simulink subsystem "iLBCTransmit"  (R2024b)
settings: Solver=VariableStepAuto  StartTime=0.0  StopTime=10.0  RelTol=1e-3
values from neighbouring files (symbols this model uses):
  in = pn()    [waveform_generator_Preamble.m]
  LSF = hexToArray(LSF,1)    [Full_transmit.m]
undefined symbols (not defined in the file or in its folder): dspblkCoreblockFVToolHelper, gcbh, ilbc, ilbcMode
libraries: simulink x19, matrix_library x13, dspmtrx3 x9, dspquant2 x6, dspilbclib x5, dspstat3 x5, dspsigops x5, simulink_need_slupdate x2, audiosources x1, dsplp x1, dspsolvers x1
(part 1 of 2)
settings Model: Creator=fredr  LastModifiedBy=fredr

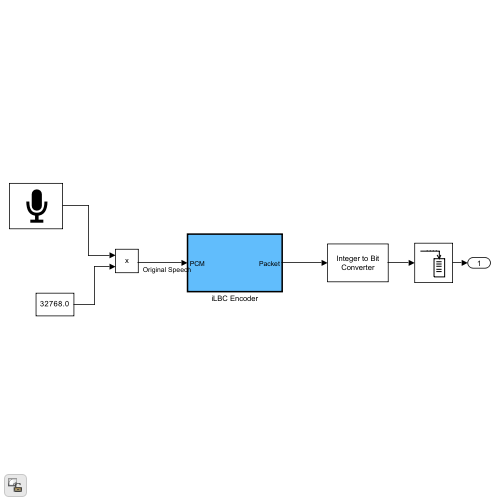
[thumbnail: Simulink's stored preview of the top-level diagram]
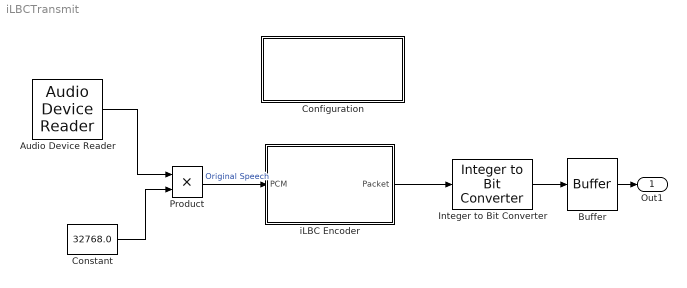
== system iLBCTransmit ==
  Audio Device Reader : audiosources/Audio Device Reader  Driver=DirectSound  Device=Default  SampleRate=8000  NumChannels=1  SamplesPerFrame=240  BitDepth=16-bit integer  NumBuffers=10  DefaultInputChannelMapping=on  InputChannelMapping=1:2  OutputNumOverrunSamples=off  OutputDataType=double  DriverIdx=1  DeviceWarnFlag=''
  Buffer : Buffer  N=200  OutputFrames=off
  Configuration : Subsystem  mask(iLBC Configuration){ilbcDialogMode=13.33 kbit/sec mode, ilbcDialogDatatype=double}
      mask prompts: ilbcDialogMode "iLBC mode:"; ilbcDialogDatatype "Internal data type:"
      mask help:
      | The iLBC standard is defined for two data rates: 13.33 kbit/sec and 15.20 kbit/sec.  Running under 13.33 kbit/sec, the encoder creates and outputs a compressed speech packet every 30ms.  With the 15.20 kbit/sec data rate, the encoder will output a packet every 20ms.  For the 13.33 kbit/sec mode, the packet size is a uint8 column vector of length 50, where each element represents one byte.  For the 15.20 kbit/sec mode, the packet is of length 38 bytes.
      |
      | The "Internal Data Type" option controls the precision for all internal floating point calculations in the iLBC Encoder and Decoder. The possible options are double and single precision.
      mask init:
      | if ilbcDialogMode == 1
      |     ilbcModeStr = '13.33';
      | elseif ilbcDialogMode == 2
      |     ilbcModeStr = '15.20';
      | end
      | 
      | if ilbcDialogDatatype == 1
      |     ilbcDatatype = 'double';
      | elseif ilbcDialogDatatype == 2
      |     ilbcDatatype = 'single';
      | end
      mask TypeOptions ilbcDialogMode: 13.33 kbit/sec mode | 15.20 kbit/sec mode
      mask TypeOptions ilbcDialogDatatype: double | single
      mask Display:
      | disp([ilbcModeStr ' kb/sec mode\n' ...
      |     'Internal data type: ' ilbcDatatype '\n' ...
      |     '[Double-click to change]']);
  Constant : Constant  Value=32768.0
  Integer to Bit Converter : simulink/Logic and Bit Operations/Integer to Bit Converter  nbits=8  signedInputValues=Unsigned  bitOrder=MSB first  outDtype=Inherit via internal rule
  Product : Product  OutDataTypeStr=int16
  iLBC Encoder : Subsystem  TreatAsAtomicUnit=on
  Out1 : Outport
  wires:
  Integer to Bit Converter/1 -> Buffer/1
  Product/1 -> iLBC Encoder/1(PCM)  "Original Speech"
  Audio Device Reader/1 -> Product/1
  iLBC Encoder/1(Packet) -> Integer to Bit Converter/1
  Buffer/1 -> Out1/1
  Constant/1 -> Product/2

== system iLBCTransmit/Configuration ==

== system iLBCTransmit/iLBC Encoder ==
  note: Section 3 of the iLBC standard
  PCM : Inport
  Calculate Residual (3.3) : Subsystem  TreatAsAtomicUnit=on
  Create Packet (3.8) : Subsystem  TreatAsAtomicUnit=on
  Data Type Conversion : DataTypeConversion  OutDataTypeStr=ilbcDatatype  SaturateOnIntegerOverflow=off  RndMeth=Floor
  Encode Data (3.5 - 3.7) : Subsystem  TreatAsAtomicUnit=on
  Encoder LPC Analysis (3.2) : Subsystem  TreatAsAtomicUnit=on
  High Pass (3.1) : DiscreteFilter  LoadFcn=dspblkCoreblockFVToolHelper(gcbh,'load');  Numerator=ilbc.hpi_zero_coefsTbl  Denominator=ilbc.hpi_pole_coefsTbl  InputProcessing=Columns as channels (frame based)  FilterStructure=Direct form II transposed  a0EqualsOne=on  NumAccumDataTypeStr=Inherit: Same as product output  DenAccumDataTypeStr=Inherit: Same as product output
      settings: CopyFcn=dspblkCoreblockFVToolHelper(gcbh,'copy');  DeleteFcn=dspblkCoreblockFVToolHelper(gcbh,'close');  ModelCloseFcn=dspblkCoreblockFVToolHelper(gcbh,'close');  PreSaveFcn=dspblkCoreblockFVToolHelper(gcbh,'presave');  PostSaveFcn=dspblkCoreblockFVToolHelper(gcbh,'postsave');  CloseFcn=dspblkCoreblockFVToolHelper(gcbh,'close');
  Perceptual Weighting (3.4) : dspmtrx3/Array-Vector Multiply  mode=Mute  saveAsFlag=0  Dimension=1  V_Source=Dialog parameter  V_VectFromMask=ilbc.LPC_CHIRP_WEIGHTDENUM.^(0:10)'  roundingMode=Floor  overflowMode=off  firstCoeffSignedness=Auto  firstCoeffDataTypeStr=Inherit: Same word length as input  firstCoeffMin=[]  firstCoeffMax=[]  firstCoeffLastDataTypeStr=Inherit: Same word length as input  prodOutputSignedness=Auto  accumSignedness=Auto  outputSignedness=Auto  outputDataTypeStr=Inherit: Same as product output  outputMin=[]  outputMax=[]  outputLastDataTypeStr=Inherit: Same as product output
  Packet : Outport  VectorParamsAs1DForOutWhenUnconnected=off
  wires:
  Encoder LPC Analysis (3.2)/2(Synthesis Filters) -> Encode Data (3.5 - 3.7)/1(Synthesis), Calculate Residual (3.3)/1(Synthesis Filters)
  Perceptual Weighting (3.4)/1 -> Encode Data (3.5 - 3.7)/2(Weights)
  PCM/1 -> Data Type Conversion/1
  Create Packet (3.8)/1(Packet) -> Packet/1
  Calculate Residual (3.3)/1(Residual) -> Encode Data (3.5 - 3.7)/3(Residual)
  Encoder LPC Analysis (3.2)/3(Weight Filters) -> Perceptual Weighting (3.4)/1
  Encode Data (3.5 - 3.7)/1(Start State Number) -> Create Packet (3.8)/2(Start State Number)
  Encode Data (3.5 - 3.7)/2(State First) -> Create Packet (3.8)/3(State First)
  Encode Data (3.5 - 3.7)/3(Start State Gain Index) -> Create Packet (3.8)/4(Start State Gain Index)
  Encode Data (3.5 - 3.7)/4(Start State Indices) -> Create Packet (3.8)/5(Start State Indices)
  Encode Data (3.5 - 3.7)/5(Code Indices) -> Create Packet (3.8)/6(Code Indices)
  Encode Data (3.5 - 3.7)/6(Gain Indices) -> Create Packet (3.8)/7(Gain Indices)
  High Pass (3.1)/1 -> Encoder LPC Analysis (3.2)/1(Data), Calculate Residual (3.3)/2(Data)
  Encoder LPC Analysis (3.2)/1(LSF Indices) -> Create Packet (3.8)/1(LSF Indices)
  Data Type Conversion/1 -> High Pass (3.1)/1

== system iLBCTransmit/iLBC Encoder/Calculate Residual (3.3) ==
  Synthesis Filters : Inport
  Data : Inport  Port=2
  Assignment1 : Assignment  NumberOfDimensions=2  OutputInitialize=Specify size for each dimension in table  IndexOptions=Assign all,Index vector (port)  Indices=-1,1  OutputSizes=40,ilbc.NSUB{ilbcMode}
  For Iterator : ForIterator  IterationLimit=ilbc.NSUB{ilbcMode}  IterationVariableDataType=int8
  Reshape2 : Reshape  OutputDimensionality=Customize  OutputDimensions=[40 ilbc.NSUB{ilbcMode}]
  Selector1 : Selector  NumberOfDimensions=2  InputPortWidth=3  IndexOptions=Select all,Index vector (port)  Indices=-1,-1  OutputSizes=1
  Selector2 : Selector  NumberOfDimensions=2  InputPortWidth=3  IndexOptions=Select all,Index vector (port)  Indices=-1,-1  OutputSizes=1
  Time-Varying Analysis Filter1 : DiscreteFir  CoefSource=Input port  Coefficients=[1 -.95]  InputProcessing=Columns as channels (frame based)  AccumDataTypeStr=Inherit: Same as product output  OutDataTypeStr=Inherit: Same as input
      settings: InputPortMap=u0,u1
  tp7f274a0e_53ba_403c_9211_c5fc596ffe5e : Math  Operator=transpose  SignedPower=on
  Residual : Outport  VectorParamsAs1DForOutWhenUnconnected=off
  wires:
  tp7f274a0e_53ba_403c_9211_c5fc596ffe5e/1 -> Time-Varying Analysis Filter1/2
  Selector1/1 -> tp7f274a0e_53ba_403c_9211_c5fc596ffe5e/1
  For Iterator/1 -> Assignment1/2, Selector2/2, Selector1/2
  Reshape2/1 -> Selector2/1
  Data/1 -> Reshape2/1
  Synthesis Filters/1 -> Selector1/1
  Assignment1/1 -> Residual/1
  Selector2/1 -> Time-Varying Analysis Filter1/1
  Time-Varying Analysis Filter1/1 -> Assignment1/1

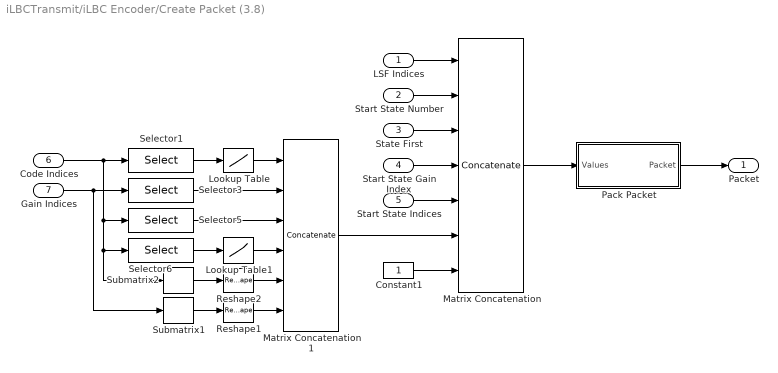
== system iLBCTransmit/iLBC Encoder/Create Packet (3.8) ==
  LSF Indices : Inport
  Start State Number : Inport  Port=2
  State First : Inport  Port=3
  Start State Gain Index : Inport  Port=4
  Start State Indices : Inport  Port=5
  Code Indices : Inport  Port=6
  Gain Indices : Inport  Port=7
  Constant1 : Constant  OutDataTypeStr=uint8
  Lookup Table : Lookup_n-D  NumberOfTableDimensions=1  BreakpointsForDimension1=[0:255]  Table=[0:57 zeros(1,70) 64:121 zeros(1,70)]  ExtrapMethod=Clip
  Lookup Table1 : Lookup_n-D  NumberOfTableDimensions=1  BreakpointsForDimension1=[0:255]  Table=[0:43 zeros(1,64) 44:107 zeros(1,64) 108:127]  ExtrapMethod=Clip
  Matrix Concatenation : Concatenate  NumInputs=7  Mode=Multidimensional array
  Matrix Concatenation1 : Concatenate  NumInputs=6  Mode=Multidimensional array
  Pack Packet : Subsystem  TreatAsAtomicUnit=on
  Reshape1 : Reshape  OutputDimensionality=Column vector (2-D)
  Reshape2 : Reshape  OutputDimensionality=Column vector (2-D)
  Selector1 : Selector  NumberOfDimensions=2  InputPortWidth=3  IndexOptions=Select all,Index vector (dialog)  Indices=-1,1  OutputSizes=1
  Selector3 : Selector  NumberOfDimensions=2  InputPortWidth=3  IndexOptions=Select all,Index vector (dialog)  Indices=-1,1  OutputSizes=1
  Selector5 : Selector  NumberOfDimensions=2  InputPortWidth=3  IndexOptions=Index vector (dialog),Index vector (dialog)  Indices=1,2  OutputSizes=1
  Selector6 : Selector  NumberOfDimensions=2  InputPortWidth=3  IndexOptions=Index vector (dialog),Index vector (dialog)  Indices=2:3,2  OutputSizes=1
  Submatrix1 : matrix_library/Submatrix  RowSpan=All rows  RowStartMode=First  RowStartIndex=1  RowEndMode=Last  RowEndIndex=1  ColSpan=Range of columns  ColStartMode=Index  ColStartIndex=2  ColEndMode=Last  ColEndIndex=1
  Submatrix2 : matrix_library/Submatrix  RowSpan=All rows  RowStartMode=First  RowStartIndex=1  RowEndMode=Last  RowEndIndex=1  ColSpan=Range of columns  ColStartMode=Index  ColStartIndex=3  ColEndMode=Last  ColEndIndex=1
  Packet : Outport  VectorParamsAs1DForOutWhenUnconnected=off
  wires:
  LSF Indices/1 -> Matrix Concatenation/1
  Start State Number/1 -> Matrix Concatenation/2
  State First/1 -> Matrix Concatenation/3
  Start State Gain Index/1 -> Matrix Concatenation/4
  Start State Indices/1 -> Matrix Concatenation/5
  Constant1/1 -> Matrix Concatenation/7
  Code Indices/1 -> Selector1/1, Selector5/1, Selector6/1, Submatrix2/1
  Selector1/1 -> Lookup Table/1
  Matrix Concatenation1/1 -> Matrix Concatenation/6
  Submatrix1/1 -> Reshape1/1
  Selector6/1 -> Lookup Table1/1
  Selector5/1 -> Matrix Concatenation1/3
  Submatrix2/1 -> Reshape2/1
  Reshape2/1 -> Matrix Concatenation1/5
  Reshape1/1 -> Matrix Concatenation1/6
  Gain Indices/1 -> Selector3/1, Submatrix1/1
  Selector3/1 -> Matrix Concatenation1/2
  Lookup Table/1 -> Matrix Concatenation1/1
  Lookup Table1/1 -> Matrix Concatenation1/4
  Matrix Concatenation/1 -> Pack Packet/1(Values)
  Pack Packet/1(Packet) -> Packet/1

== system iLBCTransmit/iLBC Encoder/Encode Data (3.5 - 3.7) ==
  Synthesis : Inport
  Weights : Inport  Port=2
  Residual : Inport  Port=3
  Decode Start State (3.5.3 last paragraph) : dspilbclib/Decode Start State  SystemSampleTime=-1  VariantActivationTime=update diagram  AllowFlexibleInterface=on  Latency=0  AutoFrameSizeCalculation=off
  Encode Remaining Sub-Blocks (3.6 - 3.7) : Subsystem
  Encode Start State (3.5.2 - 3.5.3) : Subsystem  TreatAsAtomicUnit=on
  Extract Sub-Blocks (3.5.1) and Sort LPC Filters : Subsystem  TreatAsAtomicUnit=on
  Start State Number : Outport  VectorParamsAs1DForOutWhenUnconnected=off
  State First : Outport  Port=2  VectorParamsAs1DForOutWhenUnconnected=off
  Start State Gain Index : Outport  Port=3  VectorParamsAs1DForOutWhenUnconnected=off
  Start State Indices : Outport  Port=4  VectorParamsAs1DForOutWhenUnconnected=off
  Code Indices : Outport  Port=5  VectorParamsAs1DForOutWhenUnconnected=off
  Gain Indices : Outport  Port=6  VectorParamsAs1DForOutWhenUnconnected=off
  wires:
  Extract Sub-Blocks (3.5.1) and Sort LPC Filters/4(State First) -> Encode Start State (3.5.2 - 3.5.3)/4(State First), Decode Start State (3.5.3 last paragraph)/4, State First/1, Encode Remaining Sub-Blocks (3.6 - 3.7)/4(State First)
  Residual/1 -> Extract Sub-Blocks (3.5.1) and Sort LPC Filters/1(Residual)
  Encode Start State (3.5.2 - 3.5.3)/1(Start State Indices) -> Decode Start State (3.5.3 last paragraph)/1, Start State Indices/1
  Encode Remaining Sub-Blocks (3.6 - 3.7)/1(Codes) -> Code Indices/1
  Encode Remaining Sub-Blocks (3.6 - 3.7)/2(Gains) -> Gain Indices/1
  Decode Start State (3.5.3 last paragraph)/1 -> Encode Remaining Sub-Blocks (3.6 - 3.7)/5(Initial Codebook)
  Encode Start State (3.5.2 - 3.5.3)/2(Start State Gain Index) -> Decode Start State (3.5.3 last paragraph)/2, Start State Gain Index/1
  Synthesis/1 -> Extract Sub-Blocks (3.5.1) and Sort LPC Filters/2(Synthesis)
  Extract Sub-Blocks (3.5.1) and Sort LPC Filters/1(Sorted Sub-blocks) -> Encode Remaining Sub-Blocks (3.6 - 3.7)/1(Sub-blocks)
  Extract Sub-Blocks (3.5.1) and Sort LPC Filters/2(Sorted Weights) -> Encode Remaining Sub-Blocks (3.6 - 3.7)/2(Weights)
  Weights/1 -> Extract Sub-Blocks (3.5.1) and Sort LPC Filters/3(Weights)
  Extract Sub-Blocks (3.5.1) and Sort LPC Filters/5(Start State) -> Encode Start State (3.5.2 - 3.5.3)/1(Start State)
  Extract Sub-Blocks (3.5.1) and Sort LPC Filters/6(Start State Weights) -> Encode Start State (3.5.2 - 3.5.3)/2(Weight Filters)
  Extract Sub-Blocks (3.5.1) and Sort LPC Filters/7(Start State Synthesis) -> Encode Start State (3.5.2 - 3.5.3)/3(Synthesis Filter), Decode Start State (3.5.3 last paragraph)/3
  Extract Sub-Blocks (3.5.1) and Sort LPC Filters/3(Start State Number) -> Encode Remaining Sub-Blocks (3.6 - 3.7)/3(Start State Number), Start State Number/1

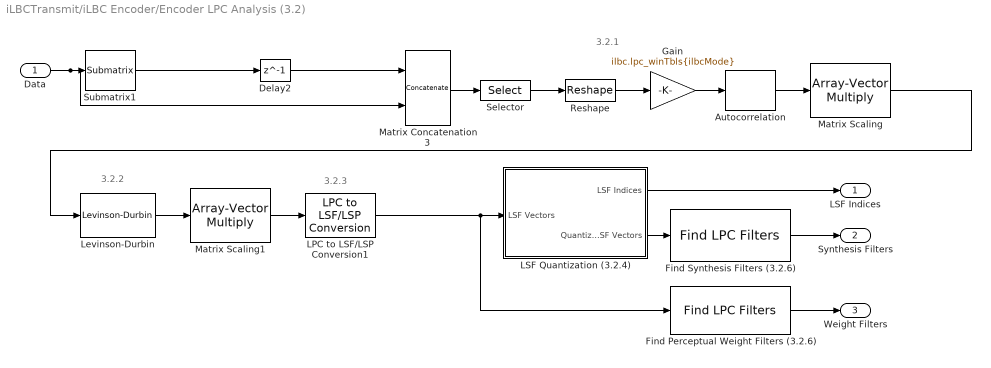
== system iLBCTransmit/iLBC Encoder/Encoder LPC Analysis (3.2) ==
  note: 3.2.3
  note: 3.2.2
  note: 3.2.1
  Data : Inport
  Autocorrelation : dspstat3/Autocorrelation  AllPositiveLags=off  maxlag=10  bias=None  domain=Time  roundingMode=Floor  overflowMode=off  outputDataTypeStr=Inherit: Same as accumulator  outputMin=[]  outputMax=[]  outputLastDataTypeStr=Inherit: Same as accumulator
  Delay2 : Delay  DelayLength=1  InitialCondition=0
  Find Perceptual Weight Filters (3.2.6) : dspilbclib/Find LPC Filters  SystemSampleTime=-1  VariantActivationTime=update diagram  AllowFlexibleInterface=on  Latency=0  AutoFrameSizeCalculation=off
  Find Synthesis Filters (3.2.6) : dspilbclib/Find LPC Filters  SystemSampleTime=-1  VariantActivationTime=update diagram  AllowFlexibleInterface=on  Latency=0  AutoFrameSizeCalculation=off
  Gain : Gain  Gain=ilbc.lpc_winTbls{ilbcMode}
  LPC to LSF/LSP Conversion1 : dsplp/LPC to LSF//LSP Conversion  output=LSF in range (0 pi)  NSteps=64  NBisects=6  RootStatus=off  correction=off  lastLSP=off  lspvector=[]  error=Ignore
  LSF Quantization (3.2.4) : Subsystem
  Levinson-Durbin : dspsolvers/Levinson-Durbin  coeffOutFcn=OBSOLETE  coeffOutFcnActive=A  outP=off  zeroInpHandling=on  roundingMode=Floor  overflowMode=off  prodOutputMode=Binary point scaling  prodOutputWordLength=32  prodOutputFracLength=30  prodOutputDataTypeStr=fixdt(1,32,30)  prodOutputLastDataTypeStr=fixdt(1,32,30)  accumMode=Binary point scaling  accumWordLength=32  accumFracLength=30  accumDataTypeStr=fixdt(1,32,30)  accumLastDataTypeStr=fixdt(1,32,30)  firstCoeffMode=Binary point scaling  firstCoeffWordLength=16  firstCoeffFracLength=15  firstCoeffDataTypeStr=fixdt(1,16,15)  firstCoeffMin=[]  firstCoeffMax=[]  firstCoeffLastDataTypeStr=fixdt(1,16,15)  secondCoeffMode=Binary point scaling  secondCoeffWordLength=16  secondCoeffFracLength=15  secondCoeffDataTypeStr=fixdt(1,16,15)  secondCoeffMin=[]  secondCoeffMax=[]  secondCoeffLastDataTypeStr=fixdt(1,16,15)  outputMin=[]  outputMax=[]
      settings: allowOverrides=off
  Matrix Concatenation3 : Concatenate  Mode=Multidimensional array
  Matrix Scaling : dspmtrx3/Array-Vector Multiply  mode=Mute  saveAsFlag=0  Dimension=1  V_Source=Dialog parameter  V_VectFromMask=ilbc.lpc_lagwinTbl  roundingMode=Floor  overflowMode=off  firstCoeffSignedness=Auto  firstCoeffDataTypeStr=Inherit: Same word length as input  firstCoeffMin=[]  firstCoeffMax=[]  firstCoeffLastDataTypeStr=Inherit: Same word length as input  prodOutputSignedness=Auto  accumSignedness=Auto  outputSignedness=Auto  outputDataTypeStr=Inherit: Same as product output  outputMin=[]  outputMax=[]  outputLastDataTypeStr=Inherit: Same as product output
  Matrix Scaling1 : dspmtrx3/Array-Vector Multiply  mode=Mute  saveAsFlag=0  Dimension=1  V_Source=Dialog parameter  V_VectFromMask=ilbc.LPC_CHIRP_SYNTDENUM.^(0:10)'  roundingMode=Floor  overflowMode=off  firstCoeffSignedness=Auto  firstCoeffDataTypeStr=Inherit: Same word length as input  firstCoeffMin=[]  firstCoeffMax=[]  firstCoeffLastDataTypeStr=Inherit: Same word length as input  prodOutputSignedness=Auto  accumSignedness=Auto  outputSignedness=Auto  outputDataTypeStr=Inherit: Same as product output  outputMin=[]  outputMax=[]  outputLastDataTypeStr=Inherit: Same as product output
  Reshape : Reshape  OutputDimensionality=Customize  OutputDimensions=[240 (3-ilbcMode)]
  Selector : Selector  NumberOfDimensions=2  InputPortWidth=3  IndexOptions=Index vector (dialog),Index vector (dialog)  Indices=ilbc.lpc_winIdxTbl{ilbcMode},1  OutputSizes=1,1
  Submatrix1 : matrix_library/Submatrix  RowSpan=Range of rows  RowStartMode=Offset from last  RowStartIndex=ilbc.BUFFEROVERLAP{ilbcMode}-1  RowEndMode=Last  RowEndIndex=1  ColSpan=All columns  ColStartMode=Offset from last  ColStartIndex=1  ColEndMode=Last  ColEndIndex=1
  LSF Indices : Outport  VectorParamsAs1DForOutWhenUnconnected=off
  Synthesis Filters : Outport  Port=2  VectorParamsAs1DForOutWhenUnconnected=off
  Weight Filters : Outport  Port=3  VectorParamsAs1DForOutWhenUnconnected=off
  wires:
  Submatrix1/1 -> Delay2/1
  Delay2/1 -> Matrix Concatenation3/1
  Matrix Scaling/1 -> Levinson-Durbin/1
  LPC to LSF/LSP Conversion1/1 -> Find Perceptual Weight Filters (3.2.6)/1, LSF Quantization (3.2.4)/1(LSF Vectors)
  Find Perceptual Weight Filters (3.2.6)/1 -> Weight Filters/1
  Find Synthesis Filters (3.2.6)/1 -> Synthesis Filters/1
  Matrix Scaling1/1 -> LPC to LSF/LSP Conversion1/1
  Levinson-Durbin/1 -> Matrix Scaling1/1
  Reshape/1 -> Gain/1
  LSF Quantization (3.2.4)/1(LSF Indices) -> LSF Indices/1
  Gain/1 -> Autocorrelation/1
  LSF Quantization (3.2.4)/2(Quantized LSF Vectors) -> Find Synthesis Filters (3.2.6)/1
  Autocorrelation/1 -> Matrix Scaling/1
  Selector/1 -> Reshape/1
  Data/1 -> Submatrix1/1, Matrix Concatenation3/2
  Matrix Concatenation3/1 -> Selector/1

== system iLBCTransmit/iLBC Encoder/Create Packet (3.8)/Pack Packet ==
  Values : Inport
  Bitwise Operator1 : simulink/Logic and Bit Operations/Bitwise Operator  logicop=AND  UseBitMask=on  BitMask=128  BitMaskRealWorld=Stored Integer
  Bitwise Operator2 : simulink/Logic and Bit Operations/Bitwise Operator  logicop=AND  UseBitMask=on  BitMask=64  BitMaskRealWorld=Stored Integer
  Bitwise Operator3 : simulink/Logic and Bit Operations/Bitwise Operator  logicop=AND  UseBitMask=on  BitMask=32  BitMaskRealWorld=Stored Integer
  Bitwise Operator4 : simulink/Logic and Bit Operations/Bitwise Operator  logicop=AND  UseBitMask=on  BitMask=16  BitMaskRealWorld=Stored Integer
  Bitwise Operator5 : simulink/Logic and Bit Operations/Bitwise Operator  logicop=AND  UseBitMask=on  BitMask=8  BitMaskRealWorld=Stored Integer
  Bitwise Operator6 : simulink/Logic and Bit Operations/Bitwise Operator  logicop=AND  UseBitMask=on  BitMask=4  BitMaskRealWorld=Stored Integer
  Bitwise Operator7 : simulink/Logic and Bit Operations/Bitwise Operator  logicop=AND  UseBitMask=on  BitMask=2  BitMaskRealWorld=Stored Integer
  Bitwise Operator8 : simulink/Logic and Bit Operations/Bitwise Operator  logicop=AND  UseBitMask=on  BitMask=1  BitMaskRealWorld=Stored Integer
  Compare To Constant8 : simulink/Logic and Bit Operations/Compare To Constant  relop=~=  const=0  OutDataTypeStr=boolean  ZeroCross=off
  Constant : Constant  Value=[128 64 32 16 8 4 2 1]'  VectorParams1D=off  OutDataTypeStr=uint8
  Matrix Concatenate : Concatenate  NumInputs=8  Mode=Multidimensional array
  Matrix Multiply : Product  Multiplication=Matrix(*)  OutDataTypeStr=uint8
  Reshape : Reshape  OutputDimensionality=Customize  OutputDimensions=[ilbc.NO_OF_BYTES{ilbcMode} 8]
  Selector : Selector  NumberOfDimensions=2  InputPortWidth=3  IndexOptions=Index vector (dialog),Select all  Indices=ilbc.bit_packTbl{ilbcMode},1  OutputSizes=1,1
  Packet : Outport  VectorParamsAs1DForOutWhenUnconnected=off
  wires:
  Compare To Constant8/1 -> Selector/1
  Bitwise Operator1/1 -> Matrix Concatenate/1
  Bitwise Operator2/1 -> Matrix Concatenate/2
  Bitwise Operator3/1 -> Matrix Concatenate/3
  Bitwise Operator4/1 -> Matrix Concatenate/4
  Bitwise Operator5/1 -> Matrix Concatenate/5
  Bitwise Operator6/1 -> Matrix Concatenate/6
  Bitwise Operator7/1 -> Matrix Concatenate/7
  Bitwise Operator8/1 -> Matrix Concatenate/8
  Selector/1 -> Reshape/1
  Reshape/1 -> Matrix Multiply/1
  Matrix Multiply/1 -> Packet/1
  Constant/1 -> Matrix Multiply/2
  Values/1 -> Bitwise Operator1/1, Bitwise Operator2/1, Bitwise Operator3/1, Bitwise Operator4/1, Bitwise Operator5/1, Bitwise Operator6/1, Bitwise Operator8/1, Bitwise Operator7/1
  Matrix Concatenate/1 -> Compare To Constant8/1

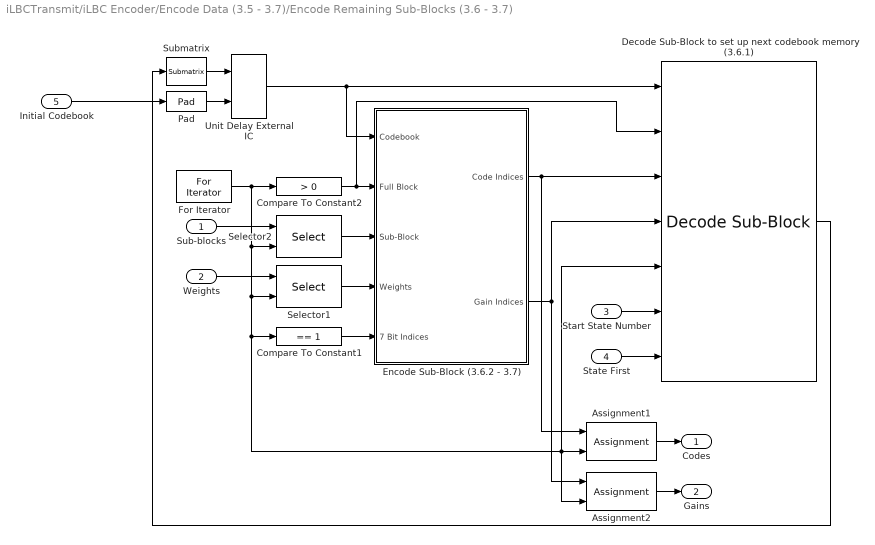
== system iLBCTransmit/iLBC Encoder/Encode Data (3.5 - 3.7)/Encode Remaining Sub-Blocks (3.6 - 3.7) ==
  Sub-blocks : Inport
  Weights : Inport  Port=2
  Start State Number : Inport  Port=3
  State First : Inport  Port=4
  Initial Codebook : Inport  Port=5
  Assignment1 : Assignment  NumberOfDimensions=2  IndexMode=Zero-based  OutputInitialize=Specify size for each dimension in table  IndexOptions=Assign all,Index vector (port)  Indices=1,1  OutputSizes=3,ilbc.NSUB{ilbcMode}-1
  Assignment2 : Assignment  NumberOfDimensions=2  IndexMode=Zero-based  OutputInitialize=Specify size for each dimension in table  IndexOptions=Assign all,Index vector (port)  Indices=1,1  OutputSizes=3,ilbc.NSUB{ilbcMode}-1
  Compare To Constant1 : simulink/Logic and Bit Operations/Compare To Constant  relop===  const=1  OutDataTypeStr=uint8  ZeroCross=off
  Compare To Constant2 : simulink/Logic and Bit Operations/Compare To Constant  relop=>  const=0  OutDataTypeStr=uint8  ZeroCross=off
  Decode Sub-Block to set up next codebook memory (3.6.1) : dspilbclib/Decode Sub-Block  SystemSampleTime=-1  VariantActivationTime=update diagram  AllowFlexibleInterface=on  Latency=0  AutoFrameSizeCalculation=off
  Encode Sub-Block (3.6.2 - 3.7) : Subsystem  TreatAsAtomicUnit=on
  For Iterator : ForIterator  ResetStates=reset  IterationLimit=ilbc.NSUB{ilbcMode}-1  IndexMode=Zero-based
  Pad : dspsigops/Pad  padAlong=Columns  dimsToPad=1  valSrc=Specify via dialog  padVal=0  spec=Pad size  padNumOutRowsSpecMethod=User-specified  numOutRows=ilbc.BLOCKL{ilbcMode}-40  padNumOutColsSpecMethod=User-specified  numOutCols=1  isVarDimsMode=off  padBeginning=90  padEnd=0  outSizeMode=User-specified  outSize=1  padSigAt=Beginning  trunc_flag=None  roundingMode=Floor  overflowMode=off  truncOrWrapMode=Truncate  wrap_flag=None
  Selector1 : Selector  NumberOfDimensions=2  IndexMode=Zero-based  InputPortWidth=3  IndexOptions=Select all,Index vector (port)  Indices=-1,0  OutputSizes=1
  Selector2 : Selector  NumberOfDimensions=2  IndexMode=Zero-based  InputPortWidth=3  IndexOptions=Select all,Index vector (port)  Indices=-1,0  OutputSizes=1
  Submatrix : matrix_library/Submatrix  RowSpan=Range of rows  RowStartMode=Index  RowStartIndex=41  RowEndMode=Last  RowEndIndex=1  ColSpan=All columns  ColStartMode=First  ColStartIndex=1  ColEndMode=Last  ColEndIndex=1
  Unit Delay External IC : simulink_need_slupdate/Unit Delay External IC  tsamp=-1
  Codes : Outport  VectorParamsAs1DForOutWhenUnconnected=off
  Gains : Outport  Port=2  VectorParamsAs1DForOutWhenUnconnected=off
  wires:
  State First/1 -> Decode Sub-Block to set up next codebook memory (3.6.1)/7
  Start State Number/1 -> Decode Sub-Block to set up next codebook memory (3.6.1)/6
  Pad/1 -> Unit Delay External IC/2
  Submatrix/1 -> Unit Delay External IC/1
  Selector2/1 -> Encode Sub-Block (3.6.2 - 3.7)/3(Sub-Block)
  Selector1/1 -> Encode Sub-Block (3.6.2 - 3.7)/4(Weights)
  Compare To Constant1/1 -> Encode Sub-Block (3.6.2 - 3.7)/5(7 Bit Indices)
  Sub-blocks/1 -> Selector2/1
  Weights/1 -> Selector1/1
  Assignment1/1 -> Codes/1
  Assignment2/1 -> Gains/1
  Unit Delay External IC/1 -> Decode Sub-Block to set up next codebook memory (3.6.1)/1, Encode Sub-Block (3.6.2 - 3.7)/1(Codebook)
  For Iterator/1 -> Selector1/2, Compare To Constant1/1, Decode Sub-Block to set up next codebook memory (3.6.1)/5, Assignment1/2, Assignment2/2, Selector2/2, Compare To Constant2/1
  Initial Codebook/1 -> Pad/1
  Decode Sub-Block to set up next codebook memory (3.6.1)/1 -> Submatrix/1
  Compare To Constant2/1 -> Decode Sub-Block to set up next codebook memory (3.6.1)/2, Encode Sub-Block (3.6.2 - 3.7)/2(Full Block)
  Encode Sub-Block (3.6.2 - 3.7)/1(Code Indices) -> Decode Sub-Block to set up next codebook memory (3.6.1)/3, Assignment1/1
  Encode Sub-Block (3.6.2 - 3.7)/2(Gain Indices) -> Decode Sub-Block to set up next codebook memory (3.6.1)/4, Assignment2/1

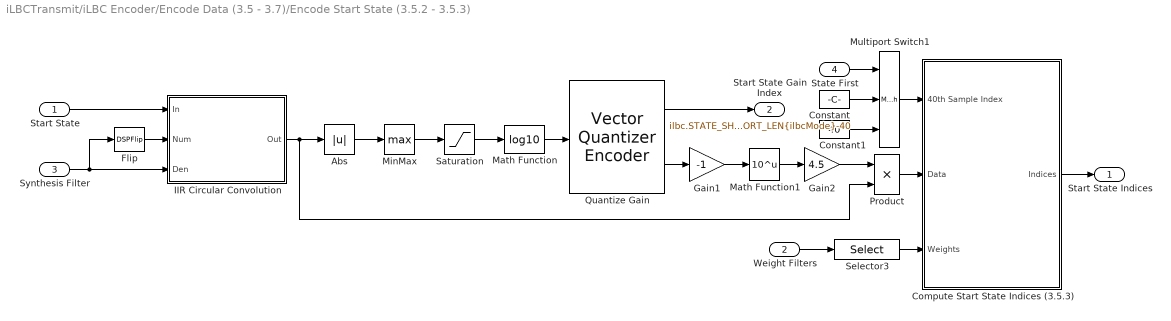
== system iLBCTransmit/iLBC Encoder/Encode Data (3.5 - 3.7)/Encode Start State (3.5.2 - 3.5.3) ==
  Start State : Inport
  Weight Filters : Inport  Port=2
  Synthesis Filter : Inport  Port=3
  State First : Inport  Port=4
  Abs : Abs  SaturateOnIntegerOverflow=off
  Compute Start State Indices (3.5.3) : Subsystem  TreatAsAtomicUnit=on
  Constant : Constant  Value=ilbc.STATE_SHORT_LEN{ilbcMode}-40  OutDataTypeStr=Inherit: Inherit via back propagation
  Constant1 : Constant  Value=40  OutDataTypeStr=Inherit: Inherit via back propagation
  Flip : DSPFlip
  Gain1 : Gain  Gain=-1  ParamDataTypeStr=Inherit: Same as input
  Gain2 : Gain  Gain=4.5  ParamDataTypeStr=Inherit: Same as input
  IIR Circular Convolution : Subsystem  TreatAsAtomicUnit=on
  Math Function : Math  Operator=log10  SignedPower=on
  Math Function1 : Math  Operator=10^u  SignedPower=on
  MinMax : MinMax  Function=max
  Multiport Switch1 : MultiPortSwitch  DataPortOrder=Zero-based contiguous  Inputs=2  zeroidx=on  SaturateOnIntegerOverflow=off  InputSameDT=off
  Product : Product  RndMeth=Zero
  Quantize Gain : dspquant2/Vector Quantizer Encoder  CBsource=Specify via dialog  codebook=ilbc.state_frgqTbl  distMeasure=Squared error  wgtSrc=Input port  weights=[1 1 1]  tieBreakRule=Choose the lower index  outQU=on  outQError=off  idtype=uint8  roundingMode=Floor  overflowMode=off
      settings: additionalParams=on
  Saturation : Saturate  UpperLimit=inf  LowerLimit=10
  Selector3 : Selector  NumberOfDimensions=2  InputPortWidth=3  IndexOptions=Index vector (dialog),Select all  Indices=2:11,-1  OutputSizes=1
  Start State Indices : Outport  VectorParamsAs1DForOutWhenUnconnected=off
  Start State Gain Index : Outport  Port=2  VectorParamsAs1DForOutWhenUnconnected=off
  wires:
  Flip/1 -> IIR Circular Convolution/2(Num)
  Abs/1 -> MinMax/1
  MinMax/1 -> Saturation/1
  Quantize Gain/2 -> Gain1/1
  Synthesis Filter/1 -> Flip/1, IIR Circular Convolution/3(Den)
  Saturation/1 -> Math Function/1
  Start State/1 -> IIR Circular Convolution/1(In)
  Compute Start State Indices (3.5.3)/1(Indices) -> Start State Indices/1
  Quantize Gain/1 -> Start State Gain Index/1
  Math Function1/1 -> Gain2/1
  Math Function/1 -> Quantize Gain/1
  Selector3/1 -> Compute Start State Indices (3.5.3)/3(Weights)
  Constant/1 -> Multiport Switch1/2
  Constant1/1 -> Multiport Switch1/3
  IIR Circular Convolution/1(Out) -> Abs/1, Product/2
  Gain1/1 -> Math Function1/1
  State First/1 -> Multiport Switch1/1
  Multiport Switch1/1 -> Compute Start State Indices (3.5.3)/1(40th Sample Index)
  Weight Filters/1 -> Selector3/1
  Product/1 -> Compute Start State Indices (3.5.3)/2(Data)
  Gain2/1 -> Product/1

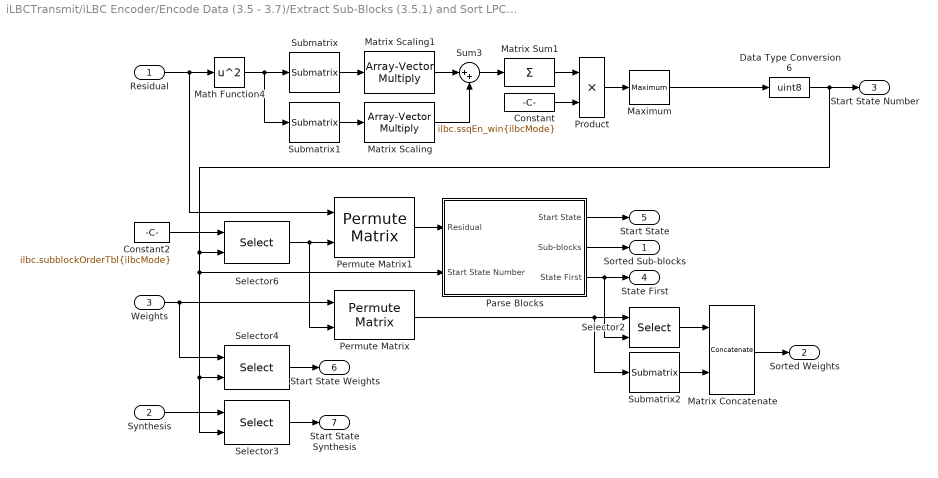
== system iLBCTransmit/iLBC Encoder/Encode Data (3.5 - 3.7)/Extract Sub-Blocks (3.5.1) and Sort LPC Filters ==
  Residual : Inport
  Synthesis : Inport  Port=2
  Weights : Inport  Port=3
  Constant : Constant  Value=ilbc.ssqEn_win{ilbcMode}  VectorParams1D=off  OutDataTypeStr=Inherit: Inherit via back propagation
  Constant2 : Constant  Value=ilbc.subblockOrderTbl{ilbcMode}  OutDataTypeStr=uint8
  Data Type Conversion6 : DataTypeConversion  OutDataTypeStr=uint8  SaturateOnIntegerOverflow=off  RndMeth=Floor
  Math Function4 : Math  Operator=square  SignedPower=on
  Matrix Concatenate : Concatenate  Mode=Multidimensional array  ConcatenateDimension=2
  Matrix Scaling : dspmtrx3/Array-Vector Multiply  mode=Mute  saveAsFlag=0  Dimension=1  V_Source=Dialog parameter  V_VectFromMask=ilbc.sampEn_win2  roundingMode=Floor  overflowMode=off  firstCoeffSignedness=Auto  firstCoeffDataTypeStr=Inherit: Same word length as input  firstCoeffMin=[]  firstCoeffMax=[]  firstCoeffLastDataTypeStr=Inherit: Same word length as input  prodOutputSignedness=Auto  accumSignedness=Auto  outputSignedness=Auto  outputMin=[]  outputMax=[]
  Matrix Scaling1 : dspmtrx3/Array-Vector Multiply  mode=Mute  saveAsFlag=0  Dimension=1  V_Source=Dialog parameter  V_VectFromMask=ilbc.sampEn_win1  roundingMode=Floor  overflowMode=off  firstCoeffSignedness=Auto  firstCoeffDataTypeStr=Inherit: Same word length as input  firstCoeffMin=[]  firstCoeffMax=[]  firstCoeffLastDataTypeStr=Inherit: Same word length as input  prodOutputSignedness=Auto  accumSignedness=Auto  outputSignedness=Auto  outputMin=[]  outputMax=[]
  Matrix Sum1 : Sum  Inputs=+  CollapseMode=Specified dimension  OutDataTypeStr=Inherit: Same as accumulator
  Maximum : dspstat3/Maximum  operation=maximum  fcn=Index  indexBase=One  operateOver=Each row  Dimension=1  InputProcessing=Columns as channels (frame based)  reset=None  roiEnable=off  roiType=Rectangles  roiPortion=Entire ROI  roiOutput=Individual statistics for each ROI  roiFlag=off  roundingMode=Floor  overflowMode=off  accumDataTypeStr=Inherit: Same as product output  accumLastDataTypeStr=Inherit: Same as product output
  Parse Blocks : Subsystem
  Permute Matrix : matrix_library/Permute Matrix  mode=Columns  ZeroOneIdxMode=One-based  errmode=Clip index  checkDims=off
  Permute Matrix1 : matrix_library/Permute Matrix  mode=Columns  ZeroOneIdxMode=One-based  errmode=Clip index  checkDims=off
  Product : Product  RndMeth=Zero
  Selector2 : Selector  NumberOfDimensions=2  IndexMode=Zero-based  InputPortWidth=3  IndexOptions=Select all,Index vector (port)  Indices=-1,1:2  OutputSizes=1
  Selector3 : Selector  NumberOfDimensions=2  InputPortWidth=3  IndexOptions=Select all,Index vector (port)  Indices=-1,-1  OutputSizes=2,2
  Selector4 : Selector  NumberOfDimensions=2  InputPortWidth=3  IndexOptions=Select all,Starting index (port)  Indices=-1,-1  OutputSizes=2,2
  Selector6 : Selector  NumberOfDimensions=2  InputPortWidth=3  IndexOptions=Index vector (port),Select all  Indices=-1,-1  OutputSizes=1
  Submatrix : matrix_library/Submatrix  RowSpan=All rows  RowStartMode=First  RowStartIndex=1  RowEndMode=Last  RowEndIndex=1  ColSpan=Range of columns  ColStartMode=First  ColStartIndex=1  ColEndMode=Offset from last  ColEndIndex=1
  Submatrix1 : matrix_library/Submatrix  RowSpan=All rows  RowStartMode=First  RowStartIndex=1  RowEndMode=Last  RowEndIndex=1  ColSpan=Range of columns  ColStartMode=Index  ColStartIndex=2  ColEndMode=Last  ColEndIndex=1
  Submatrix2 : matrix_library/Submatrix  RowSpan=All rows  RowStartMode=Index  RowStartIndex=1  RowEndMode=Last  RowEndIndex=1  ColSpan=Range of columns  ColStartMode=Index  ColStartIndex=3  ColEndMode=Last  ColEndIndex=1
  Sum3 : Sum  Inputs=|++
  Sorted Sub-blocks : Outport  VectorParamsAs1DForOutWhenUnconnected=off
  Sorted Weights : Outport  Port=2  VectorParamsAs1DForOutWhenUnconnected=off
  Start State Number : Outport  Port=3  VectorParamsAs1DForOutWhenUnconnected=off
  State First : Outport  Port=4  VectorParamsAs1DForOutWhenUnconnected=off
  Start State : Outport  Port=5  VectorParamsAs1DForOutWhenUnconnected=off
  Start State Weights : Outport  Port=6  VectorParamsAs1DForOutWhenUnconnected=off
  Start State Synthesis : Outport  Port=7  VectorParamsAs1DForOutWhenUnconnected=off
  wires:
  Parse Blocks/3(State First) -> State First/1, Selector2/2
  Parse Blocks/1(Start State) -> Start State/1
  Parse Blocks/2(Sub-blocks) -> Sorted Sub-blocks/1
  Residual/1 -> Math Function4/1, Permute Matrix1/1
  Math Function4/1 -> Submatrix/1, Submatrix1/1
  Submatrix/1 -> Matrix Scaling1/1
  Submatrix1/1 -> Matrix Scaling/1
  Matrix Scaling1/1 -> Sum3/1
  Matrix Scaling/1 -> Sum3/2
  Sum3/1 -> Matrix Sum1/1
  Matrix Sum1/1 -> Product/1
  Constant/1 -> Product/2
  Product/1 -> Maximum/1
  Maximum/1 -> Data Type Conversion6/1
  Selector3/1 -> Start State Synthesis/1
  Synthesis/1 -> Selector3/1
  Weights/1 -> Permute Matrix/1, Selector4/1
  Selector4/1 -> Start State Weights/1
  Permute Matrix/1 -> Selector2/1, Submatrix2/1
  Selector2/1 -> Matrix Concatenate/1
  Submatrix2/1 -> Matrix Concatenate/2
  Matrix Concatenate/1 -> Sorted Weights/1
  Data Type Conversion6/1 -> Start State Number/1, Parse Blocks/2(Start State Number), Selector4/2, Selector3/2, Selector6/2
  Constant2/1 -> Selector6/1
  Selector6/1 -> Permute Matrix1/2, Permute Matrix/2
  Permute Matrix1/1 -> Parse Blocks/1(Residual)

== system iLBCTransmit/iLBC Encoder/Encoder LPC Analysis (3.2)/LSF Quantization (3.2.4) ==
  LSF Vectors : Inport
  Concatenation of Quantized LSFs : Concatenate  NumInputs=3  Mode=Multidimensional array
  Concatenation of Quantized LSFs1 : Concatenate  NumInputs=3  Mode=Multidimensional array
  Reshape : Reshape  OutputDimensionality=Column vector (2-D)
  Saturation : Saturate  UpperLimit=3.14  LowerLimit=0.01
  Selector1 : Selector  NumberOfDimensions=2  InputPortWidth=3  IndexOptions=Index vector (dialog),Select all  Indices=1:3,-1  OutputSizes=1
  Selector2 : Selector  NumberOfDimensions=2  InputPortWidth=3  IndexOptions=Index vector (dialog),Select all  Indices=4:6,-1  OutputSizes=1
  Selector3 : Selector  NumberOfDimensions=2  InputPortWidth=3  IndexOptions=Index vector (dialog),Select all  Indices=7:10,-1  OutputSizes=1
  Sort : dspstat3/Sort  otype=Value  dir=Ascending  sortAlg=Quick sort  roundingMode=Floor  overflowMode=off
  VQ of LSF: 1st subvector : dspquant2/Vector Quantizer Encoder  CBsource=Specify via dialog  codebook=ilbc.lsfCbTbl1  distMeasure=Squared error  wgtSrc=Input port  weights=[1 1 1]  tieBreakRule=Choose the lower index  outQU=on  outQError=off  idtype=uint8  roundingMode=Floor  overflowMode=off
      settings: additionalParams=on
  VQ of LSF: 2nd subvector : dspquant2/Vector Quantizer Encoder  CBsource=Specify via dialog  codebook=ilbc.lsfCbTbl2  distMeasure=Squared error  wgtSrc=Input port  weights=[1 1 1]  tieBreakRule=Choose the lower index  outQU=on  outQError=off  idtype=uint8  roundingMode=Floor  overflowMode=off
      settings: additionalParams=on
  VQ of LSF: 3rd subvector : dspquant2/Vector Quantizer Encoder  CBsource=Specify via dialog  codebook=ilbc.lsfCbTbl3  distMeasure=Squared error  wgtSrc=Input port  weights=[1 1 1]  tieBreakRule=Choose the lower index  outQU=on  outQError=off  idtype=uint8  roundingMode=Floor  overflowMode=off
      settings: additionalParams=on
  LSF Indices : Outport  VectorParamsAs1DForOutWhenUnconnected=off
  Quantized LSF Vectors : Outport  Port=2  VectorParamsAs1DForOutWhenUnconnected=off
  wires:
  VQ of LSF: 1st subvector/2 -> Concatenation of Quantized LSFs/1
  VQ of LSF: 2nd subvector/2 -> Concatenation of Quantized LSFs/2
  Concatenation of Quantized LSFs/1 -> Sort/1
  VQ of LSF: 3rd subvector/2 -> Concatenation of Quantized LSFs/3
  Sort/1 -> Saturation/1
  LSF Vectors/1 -> Selector1/1, Selector3/1, Selector2/1
  Saturation/1 -> Quantized LSF Vectors/1
  Concatenation of Quantized LSFs1/1 -> Reshape/1
  VQ of LSF: 1st subvector/1 -> Concatenation of Quantized LSFs1/1
  VQ of LSF: 2nd subvector/1 -> Concatenation of Quantized LSFs1/2
  VQ of LSF: 3rd subvector/1 -> Concatenation of Quantized LSFs1/3
  Reshape/1 -> LSF Indices/1
  Selector1/1 -> VQ of LSF: 1st subvector/1
  Selector2/1 -> VQ of LSF: 2nd subvector/1
  Selector3/1 -> VQ of LSF: 3rd subvector/1

== system iLBCTransmit/iLBC Encoder/Encode Data (3.5 - 3.7)/Encode Remaining Sub-Blocks (3.6 - 3.7)/Encode Sub-Block (3.6.2 - 3.7) ==
  Codebook : Inport
  Full Block : Inport  Port=2
  Sub-Block : Inport  Port=3
  Weights : Inport  Port=4
  7 Bit Indices : Inport  Port=5
  3 Stage Sub-Block Encoder (3.6.4) : Subsystem  TreatAsAtomicUnit=on
  Adjust First Gain Index (3.7) : Subsystem  TreatAsAtomicUnit=on
  Compute Codebooks (3.6.2 - 3.6.3) : Subsystem
  Code Indices : Outport  VectorParamsAs1DForOutWhenUnconnected=off
  Gain Indices : Outport  Port=2  VectorParamsAs1DForOutWhenUnconnected=off
  wires:
  7 Bit Indices/1 -> 3 Stage Sub-Block Encoder (3.6.4)/5(7 Bit Indices)
  Full Block/1 -> 3 Stage Sub-Block Encoder (3.6.4)/6(Full Block), Compute Codebooks (3.6.2 - 3.6.3)/4(Full Block)
  Compute Codebooks (3.6.2 - 3.6.3)/4(Norms) -> 3 Stage Sub-Block Encoder (3.6.4)/4("Norms ")
  Compute Codebooks (3.6.2 - 3.6.3)/3(Augmented) -> 3 Stage Sub-Block Encoder (3.6.4)/3(Augmented)
  Compute Codebooks (3.6.2 - 3.6.3)/2(Codebooks) -> 3 Stage Sub-Block Encoder (3.6.4)/2(Codebooks)
  Compute Codebooks (3.6.2 - 3.6.3)/1(Target) -> Adjust First Gain Index (3.7)/1(Target), 3 Stage Sub-Block Encoder (3.6.4)/1(Target)
  Weights/1 -> Compute Codebooks (3.6.2 - 3.6.3)/3(Weights)
  Sub-Block/1 -> Compute Codebooks (3.6.2 - 3.6.3)/2(Sub-Block)
  Adjust First Gain Index (3.7)/1(Adjusted Gain Indices) -> Gain Indices/1
  3 Stage Sub-Block Encoder (3.6.4)/1(Code Indices) -> Code Indices/1
  3 Stage Sub-Block Encoder (3.6.4)/2(Gain Indices) -> Adjust First Gain Index (3.7)/2(Gain Indices)
  3 Stage Sub-Block Encoder (3.6.4)/3(Quantized Target) -> Adjust First Gain Index (3.7)/3(Quantized Target)
  3 Stage Sub-Block Encoder (3.6.4)/4(Quantized Gain) -> Adjust First Gain Index (3.7)/4(Quantized Gain)
  Codebook/1 -> Compute Codebooks (3.6.2 - 3.6.3)/1(Codebook)

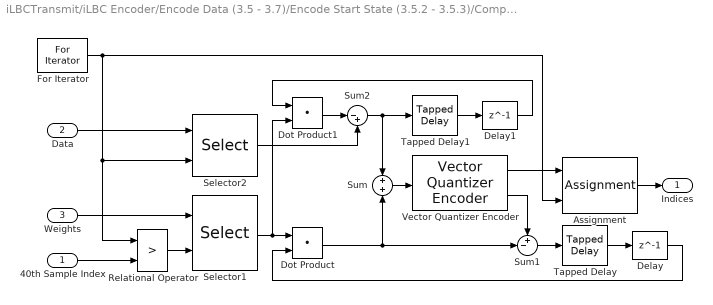
== system iLBCTransmit/iLBC Encoder/Encode Data (3.5 - 3.7)/Encode Start State (3.5.2 - 3.5.3)/Compute Start State Indices (3.5.3) ==
  40th Sample Index : Inport
  Data : Inport  Port=2
  Weights : Inport  Port=3
  Assignment : Assignment  NumberOfDimensions=2  OutputInitialize=Specify size for each dimension in table  IndexOptions=Index vector (port),Assign all  Indices=1,-1  OutputSizes=ilbc.STATE_SHORT_LEN{ilbcMode},1
  Delay : Delay  DelayLength=1  InitialCondition=0
  Delay1 : Delay  DelayLength=1  InitialCondition=0
  Dot Product : DotProduct  OutDataTypeStr=Inherit: Inherit via internal rule
  Dot Product1 : DotProduct  OutDataTypeStr=Inherit: Inherit via internal rule
  For Iterator : ForIterator  ResetStates=reset  IterationLimit=ilbc.STATE_SHORT_LEN{ilbcMode}
  Relational Operator : RelationalOperator  Operator=>  OutDataTypeStr=uint(8)  InputSameDT=off
  Selector1 : Selector  NumberOfDimensions=2  IndexMode=Zero-based  InputPortWidth=3  IndexOptions=Select all,Index vector (port)  Indices=-1,-1  OutputSizes=1
  Selector2 : Selector  NumberOfDimensions=2  InputPortWidth=3  IndexOptions=Index vector (port),Select all  Indices=-1,-1  OutputSizes=1
  Sum : Sum  Inputs=+|+  OutDataTypeStr=Inherit: Inherit via back propagation
  Sum1 : Sum  Inputs=+-|
  Sum2 : Sum  Inputs=|-+
  Tapped Delay : simulink/Discrete/Tapped Delay  vinit=0.0  samptime=-1  NumDelays=9  DelayOrder=Newest  includeCurrent=on
  Tapped Delay1 : simulink/Discrete/Tapped Delay  vinit=0.0  samptime=-1  NumDelays=9  DelayOrder=Newest  includeCurrent=on
  Vector Quantizer Encoder : dspquant2/Vector Quantizer Encoder  CBsource=Specify via dialog  codebook=ilbc.state_sq3Tbl  distMeasure=Squared error  wgtSrc=Specify via dialog  weights=[1 1 1]  tieBreakRule=Choose the lower index  outQU=on  outQError=off  idtype=uint8  roundingMode=Floor  overflowMode=on
      settings: additionalParams=on
  Indices : Outport  VectorParamsAs1DForOutWhenUnconnected=off
  wires:
  Data/1 -> Selector2/1
  Assignment/1 -> Indices/1
  40th Sample Index/1 -> Relational Operator/2
  Sum/1 -> Vector Quantizer Encoder/1
  Vector Quantizer Encoder/1 -> Assignment/1
  Vector Quantizer Encoder/2 -> Sum1/1
  Weights/1 -> Selector1/1
  Relational Operator/1 -> Selector1/2
  Selector1/1 -> Dot Product/1, Dot Product1/2
  Dot Product/1 -> Sum/2, Sum1/2
  Delay/1 -> Dot Product/2
  Tapped Delay/1 -> Delay/1
  Sum1/1 -> Tapped Delay/1
  Tapped Delay1/1 -> Delay1/1
  Sum2/1 -> Tapped Delay1/1, Sum/1
  Selector2/1 -> Sum2/2
  Delay1/1 -> Dot Product1/1
  Dot Product1/1 -> Sum2/1
  For Iterator/1 -> Relational Operator/1, Selector2/2, Assignment/2

== system iLBCTransmit/iLBC Encoder/Encode Data (3.5 - 3.7)/Encode Start State (3.5.2 - 3.5.3)/IIR Circular Convolution ==
  In : Inport
  Num : Inport  Port=2
  Den : Inport  Port=3
  Digital Filter : DiscreteFilter  NumeratorSource=Input port  Numerator=[1 2]  DenominatorSource=Input port  Denominator=[1 0.1]  InputProcessing=Columns as channels (frame based)  FilterStructure=Direct form II transposed  a0EqualsOne=on  NumAccumDataTypeStr=Inherit: Same as product output  DenAccumDataTypeStr=Inherit: Same as product output
      settings: InputPortMap=u0,p1,p3
  For Iterator : ForIterator  ResetStates=reset  IterationLimit=2  ShowIterationPort=off
  tp2c607b2c_1b80_4cca_b9d2_c4c780ba363e : Math  Operator=transpose  SignedPower=on
  tp3b2aa847_8758_4a7f_962c_1d5b50a0cc61 : Math  Operator=transpose  SignedPower=on
  Out : Outport  VectorParamsAs1DForOutWhenUnconnected=off
  wires:
  tp2c607b2c_1b80_4cca_b9d2_c4c780ba363e/1 -> Digital Filter/3
  tp3b2aa847_8758_4a7f_962c_1d5b50a0cc61/1 -> Digital Filter/2
  Den/1 -> tp2c607b2c_1b80_4cca_b9d2_c4c780ba363e/1
  Num/1 -> tp3b2aa847_8758_4a7f_962c_1d5b50a0cc61/1
  Digital Filter/1 -> Out/1
  In/1 -> Digital Filter/1

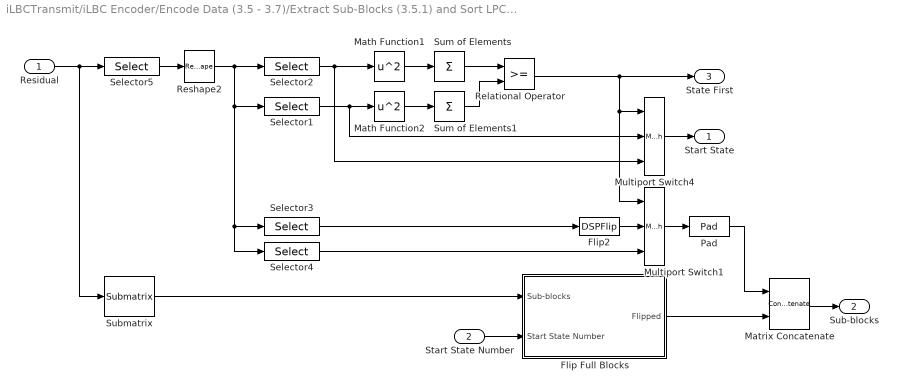
== system iLBCTransmit/iLBC Encoder/Encode Data (3.5 - 3.7)/Extract Sub-Blocks (3.5.1) and Sort LPC Filters/Parse Blocks ==
  Residual : Inport
  Start State Number : Inport  Port=2
  Flip Full Blocks : Subsystem  TreatAsAtomicUnit=on
  Flip2 : DSPFlip
  Math Function1 : Math  Operator=square  SignedPower=on
  Math Function2 : Math  Operator=square  SignedPower=on
  Matrix Concatenate : Concatenate  Mode=Multidimensional array  ConcatenateDimension=2
  Multiport Switch1 : MultiPortSwitch  DataPortOrder=Zero-based contiguous  Inputs=2  zeroidx=on  SaturateOnIntegerOverflow=off  InputSameDT=off
  Multiport Switch4 : MultiPortSwitch  DataPortOrder=Zero-based contiguous  Inputs=2  zeroidx=on  SaturateOnIntegerOverflow=off  InputSameDT=off
  Pad : dspsigops/Pad  padAlong=Columns  dimsToPad=1  valSrc=Specify via dialog  padVal=0  spec=Output size  padNumOutRowsSpecMethod=User-specified  numOutRows=40  padNumOutColsSpecMethod=User-specified  numOutCols=1  isVarDimsMode=off  padBeginning=0  padEnd=0  outSizeMode=User-specified  outSize=1  padSigAt=End  trunc_flag=None  roundingMode=Floor  overflowMode=off  truncOrWrapMode=Truncate  wrap_flag=None
  Relational Operator : RelationalOperator  OutDataTypeStr=uint(8)  InputSameDT=off
  Reshape2 : Reshape  OutputDimensionality=Column vector (2-D)
  Selector1 : Selector  NumberOfDimensions=2  InputPortWidth=3  IndexOptions=Index vector (dialog),Select all  Indices=(80-ilbc.STATE_SHORT_LEN{ilbcMode}+1):80,-1  OutputSizes=1
  Selector2 : Selector  NumberOfDimensions=2  InputPortWidth=3  IndexOptions=Index vector (dialog),Select all  Indices=1:ilbc.STATE_SHORT_LEN{ilbcMode},-1  OutputSizes=1
  Selector3 : Selector  NumberOfDimensions=2  InputPortWidth=3  IndexOptions=Starting index (dialog),Select all  Indices=1,-1  OutputSizes=80-ilbc.STATE_SHORT_LEN{ilbcMode},1
  Selector4 : Selector  NumberOfDimensions=2  InputPortWidth=3  IndexOptions=Index vector (dialog),Select all  Indices=(ilbc.STATE_SHORT_LEN{ilbcMode}+1):80,-1  OutputSizes=1
  Selector5 : Selector  NumberOfDimensions=2  InputPortWidth=3  IndexOptions=Select all,Index vector (dialog)  Indices=1:ilbc.STATE_SHORT_LEN{ilbcMode},1:2  OutputSizes=1
  Submatrix : matrix_library/Submatrix  RowSpan=All rows  RowStartMode=First  RowStartIndex=1  RowEndMode=Last  RowEndIndex=1  ColSpan=Range of columns  ColStartMode=Index  ColStartIndex=3  ColEndMode=Last  ColEndIndex=1
  Sum of Elements : Sum  Inputs=+
  Sum of Elements1 : Sum  Inputs=+
  Start State : Outport  VectorParamsAs1DForOutWhenUnconnected=off
  Sub-blocks : Outport  Port=2  VectorParamsAs1DForOutWhenUnconnected=off
  State First : Outport  Port=3  VectorParamsAs1DForOutWhenUnconnected=off
  wires:
  Selector2/1 -> Math Function1/1, Multiport Switch4/3
  Selector1/1 -> Multiport Switch4/2, Math Function2/1
  Selector4/1 -> Multiport Switch1/3
  Selector3/1 -> Flip2/1
  Sum of Elements/1 -> Relational Operator/1
  Relational Operator/1 -> Multiport Switch4/1, Multiport Switch1/1, State First/1
  Sum of Elements1/1 -> Relational Operator/2
  Math Function1/1 -> Sum of Elements/1
  Math Function2/1 -> Sum of Elements1/1
  Residual/1 -> Submatrix/1, Selector5/1
  Selector5/1 -> Reshape2/1
  Multiport Switch4/1 -> Start State/1
  Reshape2/1 -> Selector2/1, Selector1/1, Selector4/1, Selector3/1
  Multiport Switch1/1 -> Pad/1
  Pad/1 -> Matrix Concatenate/1
  Matrix Concatenate/1 -> Sub-blocks/1
  Submatrix/1 -> Flip Full Blocks/1(Sub-blocks)
  Flip Full Blocks/1(Flipped) -> Matrix Concatenate/2
  Flip2/1 -> Multiport Switch1/2
  Start State Number/1 -> Flip Full Blocks/2(Start State Number)

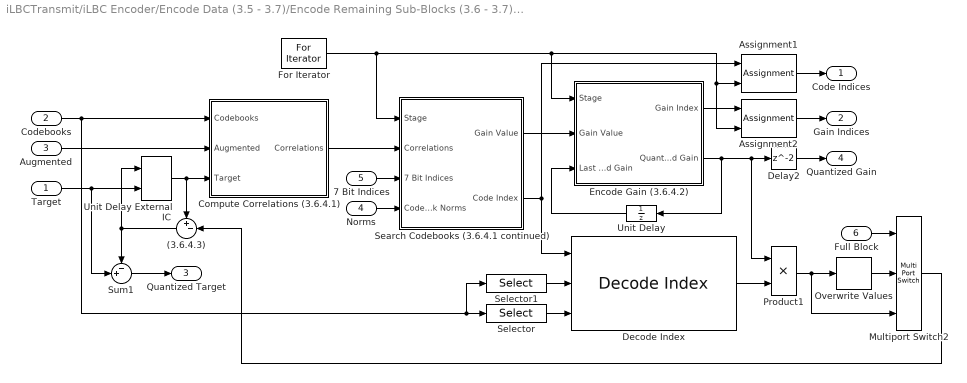
== system iLBCTransmit/iLBC Encoder/Encode Data (3.5 - 3.7)/Encode Remaining Sub-Blocks (3.6 - 3.7)/Encode Sub-Block (3.6.2 - 3.7)/3 Stage Sub-Block Encoder (3.6.4) ==
  Target : Inport
  Codebooks : Inport  Port=2
  Augmented : Inport  Port=3
  "Norms " : Inport  Port=4
  7 Bit Indices : Inport  Port=5
  Full Block : Inport  Port=6
  (3.6.4.3) : Sum  Inputs=+-|
  Assignment1 : Assignment  NumberOfDimensions=2  IndexMode=Zero-based  OutputInitialize=Specify size for each dimension in table  IndexOptions=Index vector (port),Index vector (dialog)  Indices=1,0  OutputSizes=3,1
  Assignment2 : Assignment  NumberOfDimensions=2  IndexMode=Zero-based  OutputInitialize=Specify size for each dimension in table  IndexOptions=Index vector (port),Index vector (dialog)  Indices=1,0  OutputSizes=3,1
  Compute Correlations (3.6.4.1) : Subsystem  TreatAsAtomicUnit=on
  Decode Index : dspilbclib/Decode Index  SystemSampleTime=-1  VariantActivationTime=update diagram  AllowFlexibleInterface=on  Latency=0  AutoFrameSizeCalculation=off
  Delay2 : Delay  InitialCondition=0
  Encode Gain (3.6.4.2) : Subsystem  TreatAsAtomicUnit=on
  For Iterator : ForIterator  ResetStates=reset  IterationLimit=3  IndexMode=Zero-based  IterationVariableDataType=int8
  Multiport Switch2 : MultiPortSwitch  DataPortOrder=Zero-based contiguous  Inputs=2  zeroidx=on  SaturateOnIntegerOverflow=off  InputSameDT=off
  Overwrite Values : dspmtrx3/Overwrite Values  OverWriteDiag=Submatrix  valFrom2ndIP=Specify via dialog  ConstValue=0  RowSpan=Range of rows  RowStartMode=First  RowStartIndex=1  RowEndMode=Offset from last  RowEndIndex=80-ilbc.STATE_SHORT_LEN{ilbcMode}  ColSpan=All columns  ColStartMode=First  ColStartIndex=1  ColEndMode=Last  ColEndIndex=1  DiagSpan=Range of elements  DiagStartMode=Index  DiagStartIndex=2  DiagEndMode=Index  DiagEndIndex=4
  Product1 : Product  RndMeth=Zero
  Search Codebooks (3.6.4.1 continued) : Subsystem  TreatAsAtomicUnit=on
  Selector : Selector  NumberOfDimensions=2  InputPortWidth=3  IndexOptions=Select all,Index vector (dialog)  Indices=[1 3],2  OutputSizes=1,1
  Selector1 : Selector  NumberOfDimensions=2  InputPortWidth=3  IndexOptions=Select all,Index vector (dialog)  Indices=[1 3],1  OutputSizes=1,1
  Sum1 : Sum  Inputs=-+|
  Unit Delay : UnitDelay  InitialCondition=1  SampleTime=-1  HasFrameUpgradeWarning=on
  Unit Delay External IC : simulink_need_slupdate/Unit Delay External IC  tsamp=-1
  Code Indices : Outport  VectorParamsAs1DForOutWhenUnconnected=off
  Gain Indices : Outport  Port=2  VectorParamsAs1DForOutWhenUnconnected=off
  Quantized Target : Outport  Port=3  VectorParamsAs1DForOutWhenUnconnected=off
  Quantized Gain : Outport  Port=4  VectorParamsAs1DForOutWhenUnconnected=off
  wires:
  Sum1/1 -> Quantized Target/1
  Unit Delay/1 -> Encode Gain (3.6.4.2)/3(Last Quantized Gain)
  Augmented/1 -> Compute Correlations (3.6.4.1)/2(Augmented)
  Compute Correlations (3.6.4.1)/1(Correlations) -> Search Codebooks (3.6.4.1 continued)/2(Correlations)
  Search Codebooks (3.6.4.1 continued)/2(Code Index) -> Assignment1/1, Decode Index/1
  Delay2/1 -> Quantized Gain/1
  Target/1 -> Unit Delay External IC/2, Sum1/2
  Decode Index/1 -> Product1/2
  Assignment1/1 -> Code Indices/1
  Assignment2/1 -> Gain Indices/1
  For Iterator/1 -> Search Codebooks (3.6.4.1 continued)/1(Stage), Encode Gain (3.6.4.2)/1(Stage), Assignment2/2, Assignment1/2
  (3.6.4.3)/1 -> Unit Delay External IC/1, Sum1/1
  7 Bit Indices/1 -> Search Codebooks (3.6.4.1 continued)/3(7 Bit Indices)
  "Norms "/1 -> Search Codebooks (3.6.4.1 continued)/4(Codebook Norms)
  Search Codebooks (3.6.4.1 continued)/1(Gain Value) -> Encode Gain (3.6.4.2)/2(Gain Value)
  Encode Gain (3.6.4.2)/2(Quantized Gain) -> Unit Delay/1, Delay2/1, Product1/1
  Encode Gain (3.6.4.2)/1(Gain Index) -> Assignment2/1
  Unit Delay External IC/1 -> (3.6.4.3)/1, Compute Correlations (3.6.4.1)/3(Target)
  Overwrite Values/1 -> Multiport Switch2/2
  Full Block/1 -> Multiport Switch2/1
  Selector1/1 -> Decode Index/2
  Selector/1 -> Decode Index/3
  Codebooks/1 -> Compute Correlations (3.6.4.1)/1(Codebooks), Selector/1, Selector1/1
  Product1/1 -> Overwrite Values/1, Multiport Switch2/3
  Multiport Switch2/1 -> (3.6.4.3)/2
